simulink model "assignment_2_simulink_q15"  (R2023a)
settings: Solver=VariableStepAuto  StartTime=0.0  StopTime=0.5  MaxStep=1e-6  RelTol=1e-3
libraries: simulink x1
settings Model: Creator=chowd  LastModifiedBy=chowd
settings DataIOCC: ReturnWorkspaceOutputs=off

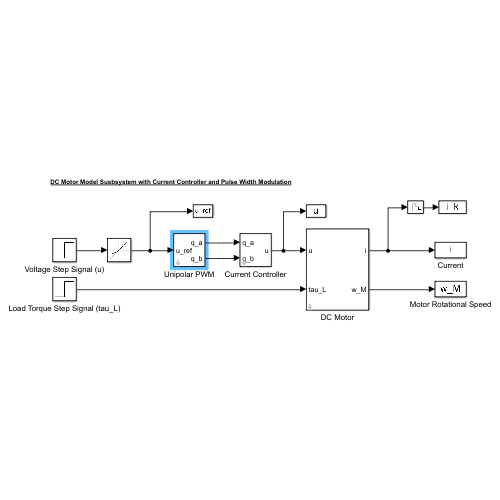
[thumbnail: Simulink's stored preview of the top-level diagram]
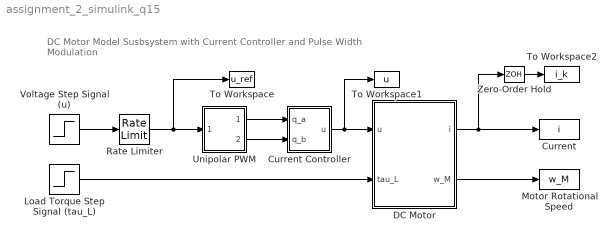
== system assignment_2_simulink_q15 ==
  note: DC Motor Model Susbsystem with Current Controller and Pulse Width Modulation
  Current : ToWorkspace  VariableName=i  SaveFormat=Timeseries  SampleTime=-1
  Current Controller : Subsystem  mask{U_dc=140}
      mask prompts: U_dc "U_dc (V)"
  DC Motor : Subsystem  mask{R=0.5, L=2.5e-3, k=0.35, J=1e-3}
      mask prompts: R "R (ohm)"; L "L (H)"; k "k (Vs)"; J "J (kgm^2)"
  Load Torque Step Signal (tau_L) : Step  Time=0.3  After=7  SampleTime=0.1
  Motor Rotational Speed : ToWorkspace  VariableName=w_M  SaveFormat=Timeseries  SampleTime=-1
  Rate Limiter : RateLimiter  RisingSlewLimit=120/0.1  FallingSlewLimit=-120/0.1  SampleTimeMode=inherited
  To Workspace : ToWorkspace  VariableName=u_ref  SaveFormat=Timeseries  SampleTime=-1
  To Workspace1 : ToWorkspace  VariableName=u  SaveFormat=Timeseries  SampleTime=-1
  To Workspace2 : ToWorkspace  VariableName=i_k  SaveFormat=Timeseries  SampleTime=-1
  Unipolar PWM : Subsystem  mask{U_dc=140, T_sw=200e-6}
      mask prompts: U_dc "U_dc (V)"; T_sw "T_sw (s)"
  Voltage Step Signal (u) : Step  Time=0.1  After=120  SampleTime=T_sw/2  mask{T_sw=200e-6}
      mask prompts: T_sw "T_sw (s)"
  Zero-Order Hold : ZeroOrderHold  SampleTime=-1
  wires:
  DC Motor/1(i) -> Current/1, Zero-Order Hold/1
  DC Motor/2(w_M) -> Motor Rotational Speed/1
  Voltage Step Signal (u)/1 -> Rate Limiter/1
  Load Torque Step Signal (tau_L)/1 -> DC Motor/2(tau_L)
  Current Controller/1(u) -> To Workspace1/1, DC Motor/1(u)
  Rate Limiter/1 -> Unipolar PWM/1(u_ref), To Workspace/1
  Unipolar PWM/1(q_a) -> Current Controller/1(q_a)
  Unipolar PWM/2(q_b) -> Current Controller/2(q_b)
  Zero-Order Hold/1 -> To Workspace2/1

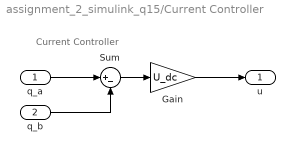
== system assignment_2_simulink_q15/Current Controller ==
  note: Current Controller
  q_a : Inport
  q_b : Inport  Port=2
  Gain : Gain  Gain=U_dc
  Sum : Sum  Inputs=|+-
  u : Outport
  wires:
  Sum/1 -> Gain/1
  Gain/1 -> u/1
  q_b/1 -> Sum/2
  q_a/1 -> Sum/1

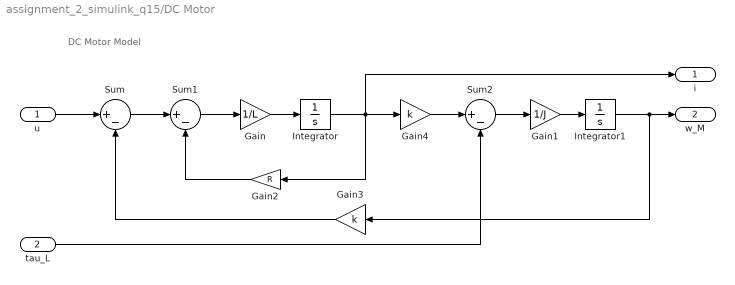
== system assignment_2_simulink_q15/DC Motor ==
  note: DC Motor Model
  u : Inport
  tau_L : Inport  Port=2
  Gain : Gain  Gain=1/L
  Gain1 : Gain  Gain=1/J
  Gain2 : Gain  Gain=R
  Gain3 : Gain  Gain=k
  Gain4 : Gain  Gain=k
  Integrator : Integrator
  Integrator1 : Integrator
  Sum : Sum  Inputs=|+-
  Sum1 : Sum  Inputs=|+-
  Sum2 : Sum  Inputs=|+-
  i : Outport
  w_M : Outport  Port=2
  wires:
  Gain/1 -> Integrator/1
  Sum2/1 -> Gain1/1
  Sum/1 -> Sum1/1
  u/1 -> Sum/1
  Integrator/1 -> Gain2/1, i/1, Gain4/1
  Sum1/1 -> Gain/1
  Gain2/1 -> Sum1/2
  Gain3/1 -> Sum/2
  tau_L/1 -> Sum2/2
  Integrator1/1 -> w_M/1, Gain3/1
  Gain4/1 -> Sum2/1
  Gain1/1 -> Integrator1/1

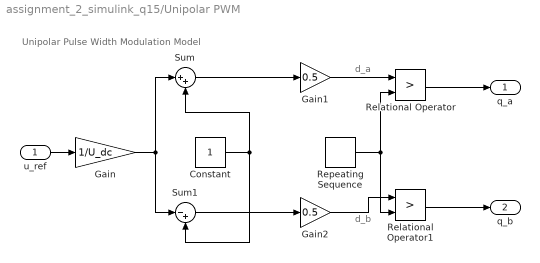
== system assignment_2_simulink_q15/Unipolar PWM ==
  note: d_a
  note: Unipolar Pulse Width Modulation Model
  note: d_b
  u_ref : Inport
  Constant : Constant
  Gain : Gain  Gain=1/U_dc
  Gain1 : Gain  Gain=0.5
  Gain2 : Gain  Gain=0.5
  Relational Operator : RelationalOperator  Operator=>  OutDataTypeStr=boolean  RndMeth=Simplest  InputSameDT=off
  Relational Operator1 : RelationalOperator  Operator=>  OutDataTypeStr=boolean  RndMeth=Simplest  InputSameDT=off
  Repeating Sequence : simulink/Sources/Repeating Sequence  rep_seq_t=T_sw*[0 0.5 1]  rep_seq_y=[1 0 1]
  Sum : Sum  Inputs=|++
  Sum1 : Sum  Inputs=|-+
  q_a : Outport
  q_b : Outport  Port=2
  wires:
  Sum1/1 -> Gain2/1
  Sum/1 -> Gain1/1
  Gain/1 -> Sum1/1, Sum/1
  u_ref/1 -> Gain/1
  Repeating Sequence/1 -> Relational Operator/2, Relational Operator1/2
  Relational Operator1/1 -> q_b/1
  Constant/1 -> Sum1/2, Sum/2
  Gain1/1 -> Relational Operator/1
  Gain2/1 -> Relational Operator1/1
  Relational Operator/1 -> q_a/1
